simulink model "TST_Rail_SetPoint"  (R2016b)
settings: Solver=FixedStepDiscrete  StartTime=0.0  StopTime=simTime  FixedStep=sampleTime  RelTol=1e-3
values from neighbouring files (symbols this model uses):
  testCase = 1    [initTST_Rail_SetPoint_001.m]    (also in initTST_Rail_SetPoint_002.m = 2)
libraries: simulink x5, UnitTest_Lib x2
settings Model: Creator=dulinggang  LastModifiedBy=dulinggang
settings DebuggingCC: SignalRangeChecking=error

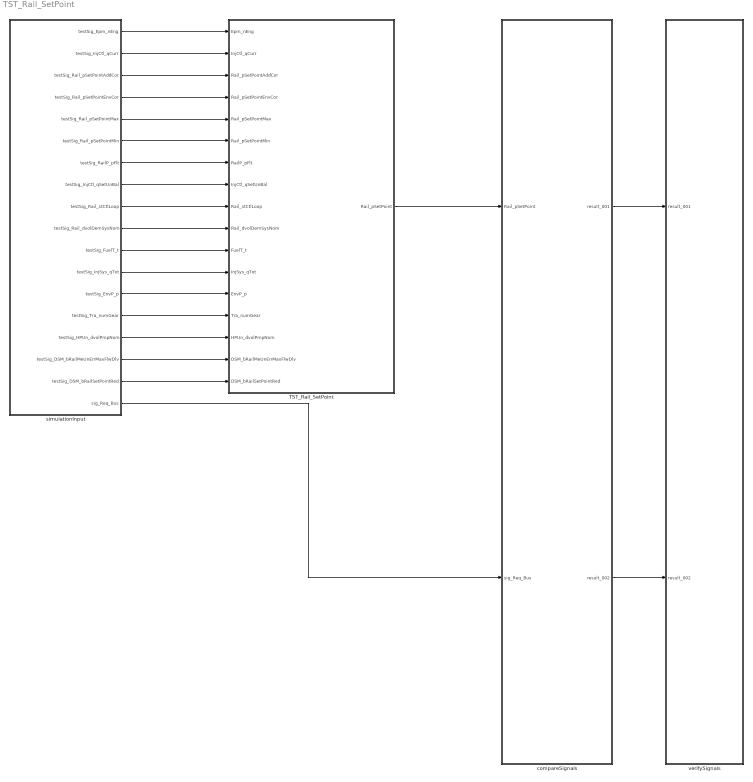
== system TST_Rail_SetPoint ==
  TST_Rail_SetPoint : Subsystem
  compareSignals : Subsystem
  simulationInput : Subsystem
  verifySignals : Subsystem
  wires:
  simulationInput/1(testSig_Epm_nEng) -> TST_Rail_SetPoint/1(Epm_nEng)
  simulationInput/2(testSig_InjCtl_qCurr) -> TST_Rail_SetPoint/2(InjCtl_qCurr)
  simulationInput/3(testSig_Rail_pSetPointAddCor) -> TST_Rail_SetPoint/3(Rail_pSetPointAddCor)
  simulationInput/4(testSig_Rail_pSetPointEnvCor) -> TST_Rail_SetPoint/4(Rail_pSetPointEnvCor)
  simulationInput/5(testSig_Rail_pSetPointMax) -> TST_Rail_SetPoint/5(Rail_pSetPointMax)
  simulationInput/6(testSig_Rail_pSetPointMin) -> TST_Rail_SetPoint/6(Rail_pSetPointMin)
  simulationInput/7(testSig_RailP_pFlt) -> TST_Rail_SetPoint/7(RailP_pFlt)
  simulationInput/8(testSig_InjCtl_qSetUnBal) -> TST_Rail_SetPoint/8(InjCtl_qSetUnBal)
  simulationInput/9(testSig_Rail_stCtlLoop) -> TST_Rail_SetPoint/9(Rail_stCtlLoop)
  simulationInput/10(testSig_Rail_dvolDemSysNom) -> TST_Rail_SetPoint/10(Rail_dvolDemSysNom)
  simulationInput/11(testSig_FuelT_t) -> TST_Rail_SetPoint/11(FuelT_t)
  simulationInput/12(testSig_InjSys_qTot) -> TST_Rail_SetPoint/12(InjSys_qTot)
  simulationInput/13(testSig_EnvP_p) -> TST_Rail_SetPoint/13(EnvP_p)
  simulationInput/14(testSig_Tra_numGear) -> TST_Rail_SetPoint/14(Tra_numGear)
  simulationInput/15(testSig_HPUn_dvolPmpNom) -> TST_Rail_SetPoint/15(HPUn_dvolPmpNom)
  simulationInput/16(testSig_DSM_bRailMeUnErrMaxFlwDlv) -> TST_Rail_SetPoint/16(DSM_bRailMeUnErrMaxFlwDlv)
  simulationInput/17(testSig_DSM_bRailSetPointRed) -> TST_Rail_SetPoint/17(DSM_bRailSetPointRed)
  TST_Rail_SetPoint/1(Rail_pSetPoint) -> compareSignals/1(Rail_pSetPoint)
  simulationInput/18(sig_Req_Bus) -> compareSignals/2(sig_Req_Bus)
  compareSignals/1(result_001) -> verifySignals/1(result_001)
  compareSignals/2(result_002) -> verifySignals/2(result_002)

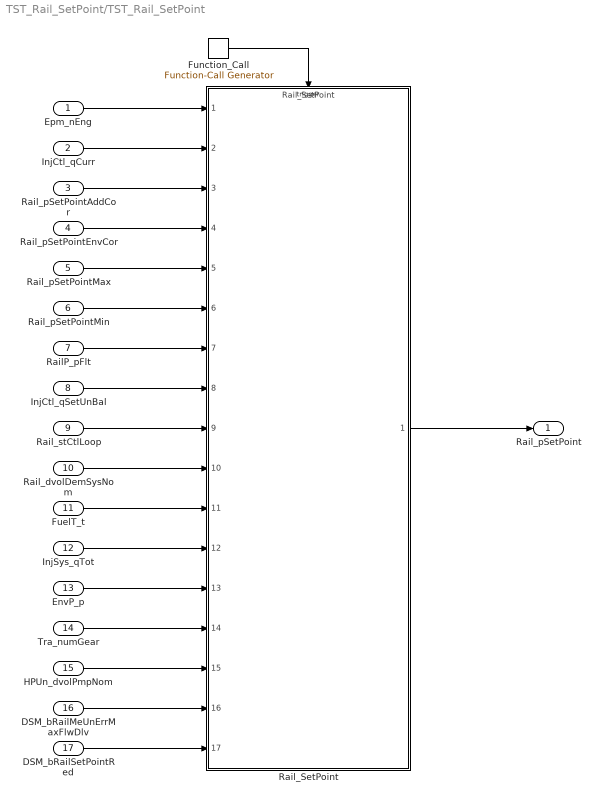
== system TST_Rail_SetPoint/TST_Rail_SetPoint ==
  Epm_nEng : Inport
  InjCtl_qCurr : Inport  Port=2
  Rail_pSetPointAddCor : Inport  Port=3
  Rail_pSetPointEnvCor : Inport  Port=4
  Rail_pSetPointMax : Inport  Port=5
  Rail_pSetPointMin : Inport  Port=6
  RailP_pFlt : Inport  Port=7
  InjCtl_qSetUnBal : Inport  Port=8
  Rail_stCtlLoop : Inport  Port=9
  Rail_dvolDemSysNom : Inport  Port=10
  FuelT_t : Inport  Port=11
  InjSys_qTot : Inport  Port=12
  EnvP_p : Inport  Port=13
  Tra_numGear : Inport  Port=14
  HPUn_dvolPmpNom : Inport  Port=15
  DSM_bRailMeUnErrMaxFlwDlv : Inport  Port=16
  DSM_bRailSetPointRed : Inport  Port=17
  Function_Call : simulink/Ports & Subsystems/Function-Call Generator  sample_time=sampleTime  numberOfIterations=1
  Rail_SetPoint : ModelReference  ModelNameDialog=Rail_SetPoint  SimulationMode=Normal  ModelReferenceVersion=1.69  TriggerPortName=function  TriggerPortTriggerType=function-call  TriggerPortStatesWhenEnabling=held
  Rail_pSetPoint : Outport
  wires:
  Function_Call/1 -> Rail_SetPoint/Trigger
  Epm_nEng/1 -> Rail_SetPoint/1
  InjCtl_qCurr/1 -> Rail_SetPoint/2
  Rail_pSetPointAddCor/1 -> Rail_SetPoint/3
  Rail_pSetPointEnvCor/1 -> Rail_SetPoint/4
  Rail_pSetPointMax/1 -> Rail_SetPoint/5
  Rail_pSetPointMin/1 -> Rail_SetPoint/6
  RailP_pFlt/1 -> Rail_SetPoint/7
  InjCtl_qSetUnBal/1 -> Rail_SetPoint/8
  Rail_stCtlLoop/1 -> Rail_SetPoint/9
  Rail_dvolDemSysNom/1 -> Rail_SetPoint/10
  FuelT_t/1 -> Rail_SetPoint/11
  InjSys_qTot/1 -> Rail_SetPoint/12
  EnvP_p/1 -> Rail_SetPoint/13
  Tra_numGear/1 -> Rail_SetPoint/14
  HPUn_dvolPmpNom/1 -> Rail_SetPoint/15
  DSM_bRailMeUnErrMaxFlwDlv/1 -> Rail_SetPoint/16
  DSM_bRailSetPointRed/1 -> Rail_SetPoint/17
  Rail_SetPoint/1 -> Rail_pSetPoint/1

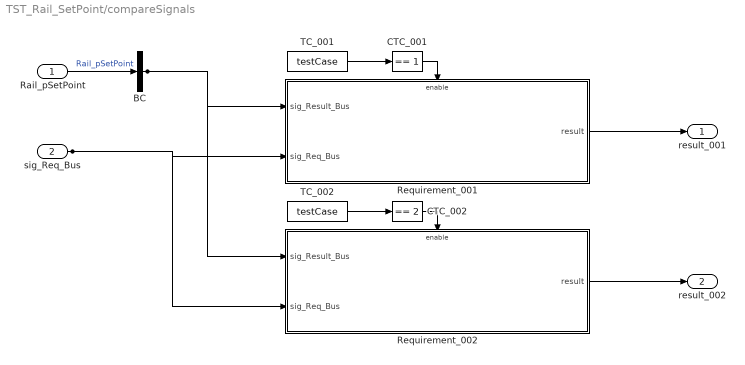
== system TST_Rail_SetPoint/compareSignals ==
  Rail_pSetPoint : Inport
  sig_Req_Bus : Inport  Port=2
  BC : BusCreator  Inputs=1
  CTC_001 : simulink/Logic and Bit Operations/Compare To Constant  relop===  const=1  OutDataTypeStr=boolean
  CTC_002 : simulink/Logic and Bit Operations/Compare To Constant  relop===  const=2  OutDataTypeStr=boolean
  Requirement_001 : Subsystem
  Requirement_002 : Subsystem
  TC_001 : Constant  Value=testCase
  TC_002 : Constant  Value=testCase
  result_001 : Outport
  result_002 : Outport  Port=2
  wires:
  Rail_pSetPoint/1 -> BC/1  "Rail_pSetPoint"
  TC_001/1 -> CTC_001/1
  CTC_001/1 -> Requirement_001/Enable
  sig_Req_Bus/1 -> Requirement_001/2(sig_Req_Bus), Requirement_002/2(sig_Req_Bus)
  BC/1 -> Requirement_001/1(sig_Result_Bus), Requirement_002/1(sig_Result_Bus)
  Requirement_001/1(result) -> result_001/1
  TC_002/1 -> CTC_002/1
  CTC_002/1 -> Requirement_002/Enable
  Requirement_002/1(result) -> result_002/1

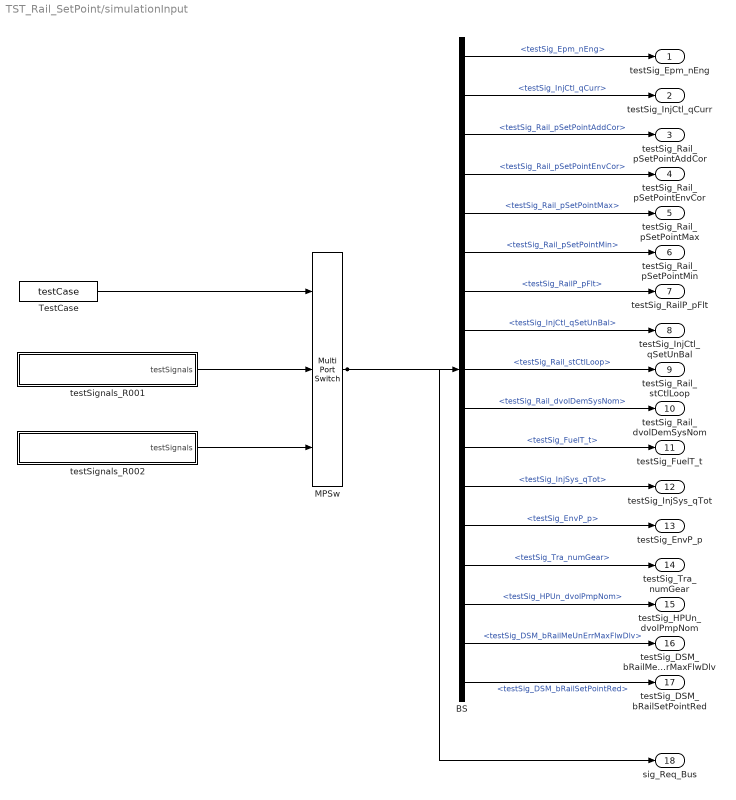
== system TST_Rail_SetPoint/simulationInput ==
  BS : BusSelector  OutputSignals=testSig_Epm_nEng,testSig_InjCtl_qCurr,testSig_Rail_pSetPointAddCor,testSig_Rail_pSetPointEnvCor,testSig_Rail_pSetPointMax,testSig_Rail_pSetPointMin,testSig_RailP_pFlt,testSig_InjCtl_qSetUnBal,testSig_Rail_stCtlLoop,testSig_Rail_dvolDemSysNom,testSig_FuelT_t,testSig_InjSys_qTot,testSig_EnvP_p,testSig_Tra_numGear,testSig_HPUn_dvolPmpNom,testSig_DSM_bRailMeUnErrMaxFlwDlv,testSig_DSM_bRailSetPointRed
  MPSw : MultiPortSwitch  Inputs=2  SaturateOnIntegerOverflow=on  InputSameDT=on
  TestCase : Constant  Value=testCase
  testSignals_R001 : Subsystem
  testSignals_R002 : Subsystem
  testSig_Epm_nEng : Outport
  testSig_InjCtl_qCurr : Outport  Port=2
  testSig_Rail_pSetPointAddCor : Outport  Port=3
  testSig_Rail_pSetPointEnvCor : Outport  Port=4
  testSig_Rail_pSetPointMax : Outport  Port=5
  testSig_Rail_pSetPointMin : Outport  Port=6
  testSig_RailP_pFlt : Outport  Port=7
  testSig_InjCtl_qSetUnBal : Outport  Port=8
  testSig_Rail_stCtlLoop : Outport  Port=9
  testSig_Rail_dvolDemSysNom : Outport  Port=10
  testSig_FuelT_t : Outport  Port=11
  testSig_InjSys_qTot : Outport  Port=12
  testSig_EnvP_p : Outport  Port=13
  testSig_Tra_numGear : Outport  Port=14
  testSig_HPUn_dvolPmpNom : Outport  Port=15
  testSig_DSM_bRailMeUnErrMaxFlwDlv : Outport  Port=16
  testSig_DSM_bRailSetPointRed : Outport  Port=17
  sig_Req_Bus : Outport  Port=18
  wires:
  BS/1 -> testSig_Epm_nEng/1  "<testSig_Epm_nEng>"
  BS/2 -> testSig_InjCtl_qCurr/1  "<testSig_InjCtl_qCurr>"
  BS/3 -> testSig_Rail_pSetPointAddCor/1  "<testSig_Rail_pSetPointAddCor>"
  BS/4 -> testSig_Rail_pSetPointEnvCor/1  "<testSig_Rail_pSetPointEnvCor>"
  BS/5 -> testSig_Rail_pSetPointMax/1  "<testSig_Rail_pSetPointMax>"
  BS/6 -> testSig_Rail_pSetPointMin/1  "<testSig_Rail_pSetPointMin>"
  BS/7 -> testSig_RailP_pFlt/1  "<testSig_RailP_pFlt>"
  BS/8 -> testSig_InjCtl_qSetUnBal/1  "<testSig_InjCtl_qSetUnBal>"
  BS/9 -> testSig_Rail_stCtlLoop/1  "<testSig_Rail_stCtlLoop>"
  BS/10 -> testSig_Rail_dvolDemSysNom/1  "<testSig_Rail_dvolDemSysNom>"
  BS/11 -> testSig_FuelT_t/1  "<testSig_FuelT_t>"
  BS/12 -> testSig_InjSys_qTot/1  "<testSig_InjSys_qTot>"
  BS/13 -> testSig_EnvP_p/1  "<testSig_EnvP_p>"
  BS/14 -> testSig_Tra_numGear/1  "<testSig_Tra_numGear>"
  BS/15 -> testSig_HPUn_dvolPmpNom/1  "<testSig_HPUn_dvolPmpNom>"
  BS/16 -> testSig_DSM_bRailMeUnErrMaxFlwDlv/1  "<testSig_DSM_bRailMeUnErrMaxFlwDlv>"
  BS/17 -> testSig_DSM_bRailSetPointRed/1  "<testSig_DSM_bRailSetPointRed>"
  MPSw/1 -> BS/1, sig_Req_Bus/1
  TestCase/1 -> MPSw/1
  testSignals_R001/1(testSignals) -> MPSw/2
  testSignals_R002/1(testSignals) -> MPSw/3

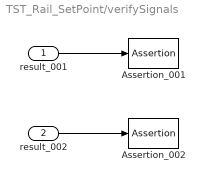
== system TST_Rail_SetPoint/verifySignals ==
  result_001 : Inport
  result_002 : Inport  Port=2
  Assertion_001 : Assertion  Enabled=off
  Assertion_002 : Assertion  Enabled=off
  wires:
  result_001/1 -> Assertion_001/1
  result_002/1 -> Assertion_002/1

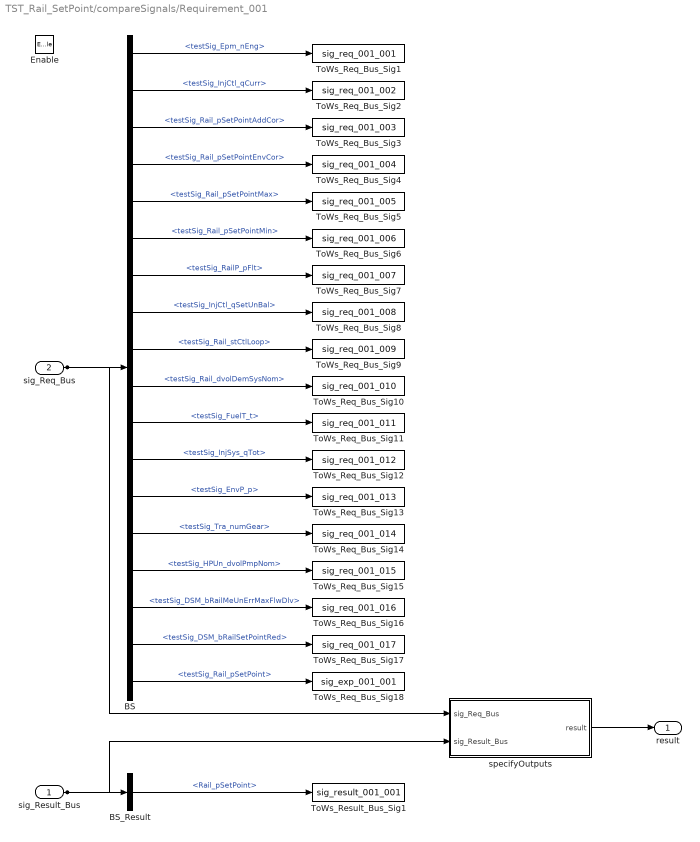
== system TST_Rail_SetPoint/compareSignals/Requirement_001 ==
  sig_Result_Bus : Inport
  sig_Req_Bus : Inport  Port=2
  Enable : EnablePort
  BS : BusSelector  OutputSignals=testSig_Epm_nEng,testSig_InjCtl_qCurr,testSig_Rail_pSetPointAddCor,testSig_Rail_pSetPointEnvCor,testSig_Rail_pSetPointMax,testSig_Rail_pSetPointMin,testSig_RailP_pFlt,testSig_InjCtl_qSetUnBal,testSig_Rail_stCtlLoop,testSig_Rail_dvolDemSysNom,testSig_FuelT_t,testSig_InjSys_qTot,testSig_EnvP_p,testSig_Tra_numGear,testSig_HPUn_dvolPmpNom,testSig_DSM_bRailMeUnErrMaxFlwDlv,testSig_DSM_bRailSetPointRed,testSig_Rail_pSetPoint
  BS_Result : BusSelector  OutputSignals=Rail_pSetPoint
  ToWs_Req_Bus_Sig1 : ToWorkspace  VariableName=sig_req_001_001  SaveFormat=Structure With Time
  ToWs_Req_Bus_Sig10 : ToWorkspace  VariableName=sig_req_001_010  SaveFormat=Structure With Time
  ToWs_Req_Bus_Sig11 : ToWorkspace  VariableName=sig_req_001_011  SaveFormat=Structure With Time
  ToWs_Req_Bus_Sig12 : ToWorkspace  VariableName=sig_req_001_012  SaveFormat=Structure With Time
  ToWs_Req_Bus_Sig13 : ToWorkspace  VariableName=sig_req_001_013  SaveFormat=Structure With Time
  ToWs_Req_Bus_Sig14 : ToWorkspace  VariableName=sig_req_001_014  SaveFormat=Structure With Time
  ToWs_Req_Bus_Sig15 : ToWorkspace  VariableName=sig_req_001_015  SaveFormat=Structure With Time
  ToWs_Req_Bus_Sig16 : ToWorkspace  VariableName=sig_req_001_016  SaveFormat=Structure With Time
  ToWs_Req_Bus_Sig17 : ToWorkspace  VariableName=sig_req_001_017  SaveFormat=Structure With Time
  ToWs_Req_Bus_Sig18 : ToWorkspace  VariableName=sig_exp_001_001  SaveFormat=Structure With Time
  ToWs_Req_Bus_Sig2 : ToWorkspace  VariableName=sig_req_001_002  SaveFormat=Structure With Time
  ToWs_Req_Bus_Sig3 : ToWorkspace  VariableName=sig_req_001_003  SaveFormat=Structure With Time
  ToWs_Req_Bus_Sig4 : ToWorkspace  VariableName=sig_req_001_004  SaveFormat=Structure With Time
  ToWs_Req_Bus_Sig5 : ToWorkspace  VariableName=sig_req_001_005  SaveFormat=Structure With Time
  ToWs_Req_Bus_Sig6 : ToWorkspace  VariableName=sig_req_001_006  SaveFormat=Structure With Time
  ToWs_Req_Bus_Sig7 : ToWorkspace  VariableName=sig_req_001_007  SaveFormat=Structure With Time
  ToWs_Req_Bus_Sig8 : ToWorkspace  VariableName=sig_req_001_008  SaveFormat=Structure With Time
  ToWs_Req_Bus_Sig9 : ToWorkspace  VariableName=sig_req_001_009  SaveFormat=Structure With Time
  ToWs_Result_Bus_Sig1 : ToWorkspace  VariableName=sig_result_001_001  SaveFormat=Structure With Time
  specifyOutputs : Subsystem
  result : Outport
  wires:
  sig_Req_Bus/1 -> BS/1, specifyOutputs/1(sig_Req_Bus)
  BS/1 -> ToWs_Req_Bus_Sig1/1  "<testSig_Epm_nEng>"
  BS/2 -> ToWs_Req_Bus_Sig2/1  "<testSig_InjCtl_qCurr>"
  BS/3 -> ToWs_Req_Bus_Sig3/1  "<testSig_Rail_pSetPointAddCor>"
  BS/4 -> ToWs_Req_Bus_Sig4/1  "<testSig_Rail_pSetPointEnvCor>"
  BS/5 -> ToWs_Req_Bus_Sig5/1  "<testSig_Rail_pSetPointMax>"
  BS/6 -> ToWs_Req_Bus_Sig6/1  "<testSig_Rail_pSetPointMin>"
  BS/7 -> ToWs_Req_Bus_Sig7/1  "<testSig_RailP_pFlt>"
  BS/8 -> ToWs_Req_Bus_Sig8/1  "<testSig_InjCtl_qSetUnBal>"
  BS/9 -> ToWs_Req_Bus_Sig9/1  "<testSig_Rail_stCtlLoop>"
  BS/10 -> ToWs_Req_Bus_Sig10/1  "<testSig_Rail_dvolDemSysNom>"
  BS/11 -> ToWs_Req_Bus_Sig11/1  "<testSig_FuelT_t>"
  BS/12 -> ToWs_Req_Bus_Sig12/1  "<testSig_InjSys_qTot>"
  BS/13 -> ToWs_Req_Bus_Sig13/1  "<testSig_EnvP_p>"
  BS/14 -> ToWs_Req_Bus_Sig14/1  "<testSig_Tra_numGear>"
  BS/15 -> ToWs_Req_Bus_Sig15/1  "<testSig_HPUn_dvolPmpNom>"
  BS/16 -> ToWs_Req_Bus_Sig16/1  "<testSig_DSM_bRailMeUnErrMaxFlwDlv>"
  BS/17 -> ToWs_Req_Bus_Sig17/1  "<testSig_DSM_bRailSetPointRed>"
  BS/18 -> ToWs_Req_Bus_Sig18/1  "<testSig_Rail_pSetPoint>"
  sig_Result_Bus/1 -> BS_Result/1, specifyOutputs/2(sig_Result_Bus)
  BS_Result/1 -> ToWs_Result_Bus_Sig1/1  "<Rail_pSetPoint>"
  specifyOutputs/1(result) -> result/1

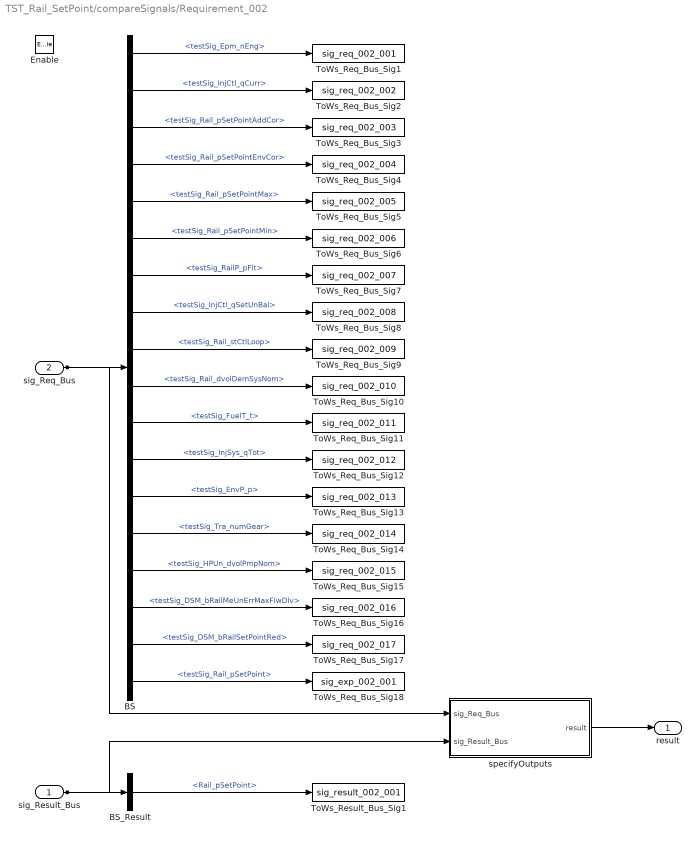
== system TST_Rail_SetPoint/compareSignals/Requirement_002 ==
  sig_Result_Bus : Inport
  sig_Req_Bus : Inport  Port=2
  Enable : EnablePort
  BS : BusSelector  OutputSignals=testSig_Epm_nEng,testSig_InjCtl_qCurr,testSig_Rail_pSetPointAddCor,testSig_Rail_pSetPointEnvCor,testSig_Rail_pSetPointMax,testSig_Rail_pSetPointMin,testSig_RailP_pFlt,testSig_InjCtl_qSetUnBal,testSig_Rail_stCtlLoop,testSig_Rail_dvolDemSysNom,testSig_FuelT_t,testSig_InjSys_qTot,testSig_EnvP_p,testSig_Tra_numGear,testSig_HPUn_dvolPmpNom,testSig_DSM_bRailMeUnErrMaxFlwDlv,testSig_DSM_bRailSetPointRed,testSig_Rail_pSetPoint
  BS_Result : BusSelector  OutputSignals=Rail_pSetPoint
  ToWs_Req_Bus_Sig1 : ToWorkspace  VariableName=sig_req_002_001  SaveFormat=Structure With Time
  ToWs_Req_Bus_Sig10 : ToWorkspace  VariableName=sig_req_002_010  SaveFormat=Structure With Time
  ToWs_Req_Bus_Sig11 : ToWorkspace  VariableName=sig_req_002_011  SaveFormat=Structure With Time
  ToWs_Req_Bus_Sig12 : ToWorkspace  VariableName=sig_req_002_012  SaveFormat=Structure With Time
  ToWs_Req_Bus_Sig13 : ToWorkspace  VariableName=sig_req_002_013  SaveFormat=Structure With Time
  ToWs_Req_Bus_Sig14 : ToWorkspace  VariableName=sig_req_002_014  SaveFormat=Structure With Time
  ToWs_Req_Bus_Sig15 : ToWorkspace  VariableName=sig_req_002_015  SaveFormat=Structure With Time
  ToWs_Req_Bus_Sig16 : ToWorkspace  VariableName=sig_req_002_016  SaveFormat=Structure With Time
  ToWs_Req_Bus_Sig17 : ToWorkspace  VariableName=sig_req_002_017  SaveFormat=Structure With Time
  ToWs_Req_Bus_Sig18 : ToWorkspace  VariableName=sig_exp_002_001  SaveFormat=Structure With Time
  ToWs_Req_Bus_Sig2 : ToWorkspace  VariableName=sig_req_002_002  SaveFormat=Structure With Time
  ToWs_Req_Bus_Sig3 : ToWorkspace  VariableName=sig_req_002_003  SaveFormat=Structure With Time
  ToWs_Req_Bus_Sig4 : ToWorkspace  VariableName=sig_req_002_004  SaveFormat=Structure With Time
  ToWs_Req_Bus_Sig5 : ToWorkspace  VariableName=sig_req_002_005  SaveFormat=Structure With Time
  ToWs_Req_Bus_Sig6 : ToWorkspace  VariableName=sig_req_002_006  SaveFormat=Structure With Time
  ToWs_Req_Bus_Sig7 : ToWorkspace  VariableName=sig_req_002_007  SaveFormat=Structure With Time
  ToWs_Req_Bus_Sig8 : ToWorkspace  VariableName=sig_req_002_008  SaveFormat=Structure With Time
  ToWs_Req_Bus_Sig9 : ToWorkspace  VariableName=sig_req_002_009  SaveFormat=Structure With Time
  ToWs_Result_Bus_Sig1 : ToWorkspace  VariableName=sig_result_002_001  SaveFormat=Structure With Time
  specifyOutputs : Subsystem
  result : Outport
  wires:
  sig_Req_Bus/1 -> BS/1, specifyOutputs/1(sig_Req_Bus)
  BS/1 -> ToWs_Req_Bus_Sig1/1  "<testSig_Epm_nEng>"
  BS/2 -> ToWs_Req_Bus_Sig2/1  "<testSig_InjCtl_qCurr>"
  BS/3 -> ToWs_Req_Bus_Sig3/1  "<testSig_Rail_pSetPointAddCor>"
  BS/4 -> ToWs_Req_Bus_Sig4/1  "<testSig_Rail_pSetPointEnvCor>"
  BS/5 -> ToWs_Req_Bus_Sig5/1  "<testSig_Rail_pSetPointMax>"
  BS/6 -> ToWs_Req_Bus_Sig6/1  "<testSig_Rail_pSetPointMin>"
  BS/7 -> ToWs_Req_Bus_Sig7/1  "<testSig_RailP_pFlt>"
  BS/8 -> ToWs_Req_Bus_Sig8/1  "<testSig_InjCtl_qSetUnBal>"
  BS/9 -> ToWs_Req_Bus_Sig9/1  "<testSig_Rail_stCtlLoop>"
  BS/10 -> ToWs_Req_Bus_Sig10/1  "<testSig_Rail_dvolDemSysNom>"
  BS/11 -> ToWs_Req_Bus_Sig11/1  "<testSig_FuelT_t>"
  BS/12 -> ToWs_Req_Bus_Sig12/1  "<testSig_InjSys_qTot>"
  BS/13 -> ToWs_Req_Bus_Sig13/1  "<testSig_EnvP_p>"
  BS/14 -> ToWs_Req_Bus_Sig14/1  "<testSig_Tra_numGear>"
  BS/15 -> ToWs_Req_Bus_Sig15/1  "<testSig_HPUn_dvolPmpNom>"
  BS/16 -> ToWs_Req_Bus_Sig16/1  "<testSig_DSM_bRailMeUnErrMaxFlwDlv>"
  BS/17 -> ToWs_Req_Bus_Sig17/1  "<testSig_DSM_bRailSetPointRed>"
  BS/18 -> ToWs_Req_Bus_Sig18/1  "<testSig_Rail_pSetPoint>"
  sig_Result_Bus/1 -> BS_Result/1, specifyOutputs/2(sig_Result_Bus)
  BS_Result/1 -> ToWs_Result_Bus_Sig1/1  "<Rail_pSetPoint>"
  specifyOutputs/1(result) -> result/1

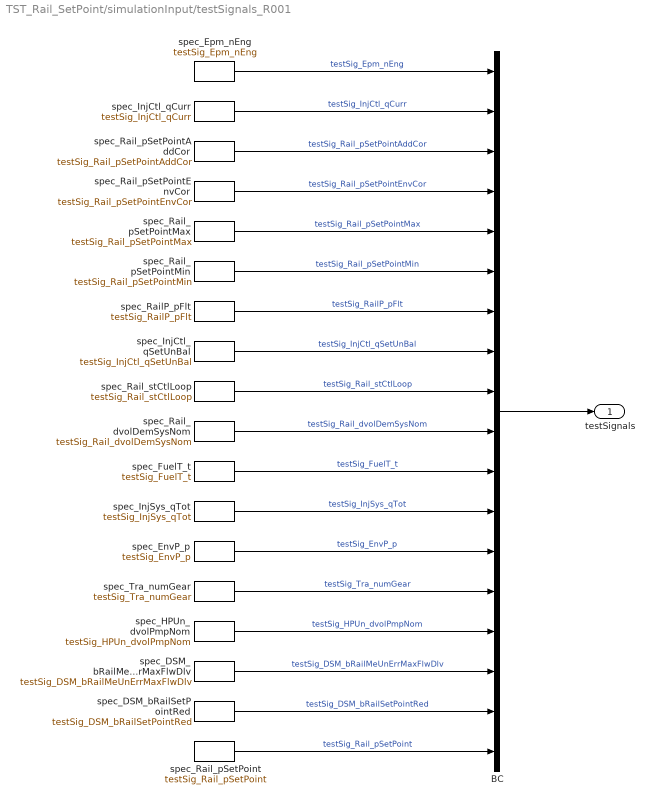
== system TST_Rail_SetPoint/simulationInput/testSignals_R001 ==
  BC : BusCreator  Inputs=18
  spec_DSM_bRailMeUnErrMaxFlwDlv : FromWorkspace  VariableName=testSig_DSM_bRailMeUnErrMaxFlwDlv  Interpolate=off  OutputAfterFinalValue=Holding final value
  spec_DSM_bRailSetPointRed : FromWorkspace  VariableName=testSig_DSM_bRailSetPointRed  Interpolate=off  OutputAfterFinalValue=Holding final value
  spec_EnvP_p : FromWorkspace  VariableName=testSig_EnvP_p  Interpolate=off  OutputAfterFinalValue=Holding final value
  spec_Epm_nEng : FromWorkspace  VariableName=testSig_Epm_nEng  Interpolate=off  OutputAfterFinalValue=Holding final value
  spec_FuelT_t : FromWorkspace  VariableName=testSig_FuelT_t  Interpolate=off  OutputAfterFinalValue=Holding final value
  spec_HPUn_dvolPmpNom : FromWorkspace  VariableName=testSig_HPUn_dvolPmpNom  Interpolate=off  OutputAfterFinalValue=Holding final value
  spec_InjCtl_qCurr : FromWorkspace  VariableName=testSig_InjCtl_qCurr  Interpolate=off  OutputAfterFinalValue=Holding final value
  spec_InjCtl_qSetUnBal : FromWorkspace  VariableName=testSig_InjCtl_qSetUnBal  Interpolate=off  OutputAfterFinalValue=Holding final value
  spec_InjSys_qTot : FromWorkspace  VariableName=testSig_InjSys_qTot  Interpolate=off  OutputAfterFinalValue=Holding final value
  spec_RailP_pFlt : FromWorkspace  VariableName=testSig_RailP_pFlt  Interpolate=off  OutputAfterFinalValue=Holding final value
  spec_Rail_dvolDemSysNom : FromWorkspace  VariableName=testSig_Rail_dvolDemSysNom  Interpolate=off  OutputAfterFinalValue=Holding final value
  spec_Rail_pSetPoint : FromWorkspace  VariableName=testSig_Rail_pSetPoint  Interpolate=off  OutputAfterFinalValue=Holding final value
  spec_Rail_pSetPointAddCor : FromWorkspace  VariableName=testSig_Rail_pSetPointAddCor  Interpolate=off  OutputAfterFinalValue=Holding final value
  spec_Rail_pSetPointEnvCor : FromWorkspace  VariableName=testSig_Rail_pSetPointEnvCor  Interpolate=off  OutputAfterFinalValue=Holding final value
  spec_Rail_pSetPointMax : FromWorkspace  VariableName=testSig_Rail_pSetPointMax  Interpolate=off  OutputAfterFinalValue=Holding final value
  spec_Rail_pSetPointMin : FromWorkspace  VariableName=testSig_Rail_pSetPointMin  Interpolate=off  OutputAfterFinalValue=Holding final value
  spec_Rail_stCtlLoop : FromWorkspace  VariableName=testSig_Rail_stCtlLoop  Interpolate=off  OutputAfterFinalValue=Holding final value
  spec_Tra_numGear : FromWorkspace  VariableName=testSig_Tra_numGear  Interpolate=off  OutputAfterFinalValue=Holding final value
  testSignals : Outport
  wires:
  BC/1 -> testSignals/1
  spec_Epm_nEng/1 -> BC/1  "testSig_Epm_nEng"
  spec_InjCtl_qCurr/1 -> BC/2  "testSig_InjCtl_qCurr"
  spec_Rail_pSetPointAddCor/1 -> BC/3  "testSig_Rail_pSetPointAddCor"
  spec_Rail_pSetPointEnvCor/1 -> BC/4  "testSig_Rail_pSetPointEnvCor"
  spec_Rail_pSetPointMax/1 -> BC/5  "testSig_Rail_pSetPointMax"
  spec_Rail_pSetPointMin/1 -> BC/6  "testSig_Rail_pSetPointMin"
  spec_RailP_pFlt/1 -> BC/7  "testSig_RailP_pFlt"
  spec_InjCtl_qSetUnBal/1 -> BC/8  "testSig_InjCtl_qSetUnBal"
  spec_Rail_stCtlLoop/1 -> BC/9  "testSig_Rail_stCtlLoop"
  spec_Rail_dvolDemSysNom/1 -> BC/10  "testSig_Rail_dvolDemSysNom"
  spec_FuelT_t/1 -> BC/11  "testSig_FuelT_t"
  spec_InjSys_qTot/1 -> BC/12  "testSig_InjSys_qTot"
  spec_EnvP_p/1 -> BC/13  "testSig_EnvP_p"
  spec_Tra_numGear/1 -> BC/14  "testSig_Tra_numGear"
  spec_HPUn_dvolPmpNom/1 -> BC/15  "testSig_HPUn_dvolPmpNom"
  spec_DSM_bRailMeUnErrMaxFlwDlv/1 -> BC/16  "testSig_DSM_bRailMeUnErrMaxFlwDlv"
  spec_DSM_bRailSetPointRed/1 -> BC/17  "testSig_DSM_bRailSetPointRed"
  spec_Rail_pSetPoint/1 -> BC/18  "testSig_Rail_pSetPoint"

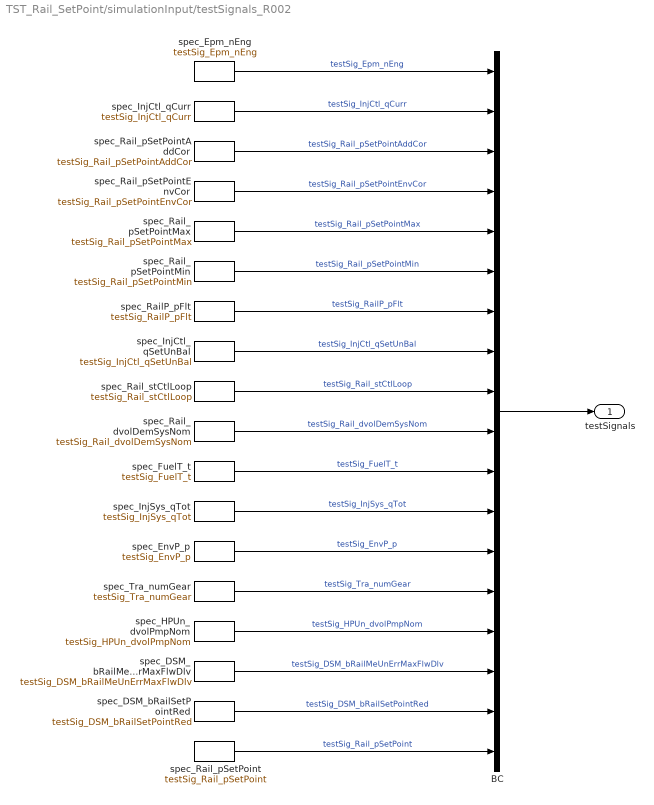
== system TST_Rail_SetPoint/simulationInput/testSignals_R002 ==
  BC : BusCreator  Inputs=18
  spec_DSM_bRailMeUnErrMaxFlwDlv : FromWorkspace  VariableName=testSig_DSM_bRailMeUnErrMaxFlwDlv  Interpolate=off  OutputAfterFinalValue=Holding final value
  spec_DSM_bRailSetPointRed : FromWorkspace  VariableName=testSig_DSM_bRailSetPointRed  Interpolate=off  OutputAfterFinalValue=Holding final value
  spec_EnvP_p : FromWorkspace  VariableName=testSig_EnvP_p  Interpolate=off  OutputAfterFinalValue=Holding final value
  spec_Epm_nEng : FromWorkspace  VariableName=testSig_Epm_nEng  Interpolate=off  OutputAfterFinalValue=Holding final value
  spec_FuelT_t : FromWorkspace  VariableName=testSig_FuelT_t  Interpolate=off  OutputAfterFinalValue=Holding final value
  spec_HPUn_dvolPmpNom : FromWorkspace  VariableName=testSig_HPUn_dvolPmpNom  Interpolate=off  OutputAfterFinalValue=Holding final value
  spec_InjCtl_qCurr : FromWorkspace  VariableName=testSig_InjCtl_qCurr  Interpolate=off  OutputAfterFinalValue=Holding final value
  spec_InjCtl_qSetUnBal : FromWorkspace  VariableName=testSig_InjCtl_qSetUnBal  Interpolate=off  OutputAfterFinalValue=Holding final value
  spec_InjSys_qTot : FromWorkspace  VariableName=testSig_InjSys_qTot  Interpolate=off  OutputAfterFinalValue=Holding final value
  spec_RailP_pFlt : FromWorkspace  VariableName=testSig_RailP_pFlt  Interpolate=off  OutputAfterFinalValue=Holding final value
  spec_Rail_dvolDemSysNom : FromWorkspace  VariableName=testSig_Rail_dvolDemSysNom  Interpolate=off  OutputAfterFinalValue=Holding final value
  spec_Rail_pSetPoint : FromWorkspace  VariableName=testSig_Rail_pSetPoint  Interpolate=off  OutputAfterFinalValue=Holding final value
  spec_Rail_pSetPointAddCor : FromWorkspace  VariableName=testSig_Rail_pSetPointAddCor  Interpolate=off  OutputAfterFinalValue=Holding final value
  spec_Rail_pSetPointEnvCor : FromWorkspace  VariableName=testSig_Rail_pSetPointEnvCor  Interpolate=off  OutputAfterFinalValue=Holding final value
  spec_Rail_pSetPointMax : FromWorkspace  VariableName=testSig_Rail_pSetPointMax  Interpolate=off  OutputAfterFinalValue=Holding final value
  spec_Rail_pSetPointMin : FromWorkspace  VariableName=testSig_Rail_pSetPointMin  Interpolate=off  OutputAfterFinalValue=Holding final value
  spec_Rail_stCtlLoop : FromWorkspace  VariableName=testSig_Rail_stCtlLoop  Interpolate=off  OutputAfterFinalValue=Holding final value
  spec_Tra_numGear : FromWorkspace  VariableName=testSig_Tra_numGear  Interpolate=off  OutputAfterFinalValue=Holding final value
  testSignals : Outport
  wires:
  BC/1 -> testSignals/1
  spec_Epm_nEng/1 -> BC/1  "testSig_Epm_nEng"
  spec_InjCtl_qCurr/1 -> BC/2  "testSig_InjCtl_qCurr"
  spec_Rail_pSetPointAddCor/1 -> BC/3  "testSig_Rail_pSetPointAddCor"
  spec_Rail_pSetPointEnvCor/1 -> BC/4  "testSig_Rail_pSetPointEnvCor"
  spec_Rail_pSetPointMax/1 -> BC/5  "testSig_Rail_pSetPointMax"
  spec_Rail_pSetPointMin/1 -> BC/6  "testSig_Rail_pSetPointMin"
  spec_RailP_pFlt/1 -> BC/7  "testSig_RailP_pFlt"
  spec_InjCtl_qSetUnBal/1 -> BC/8  "testSig_InjCtl_qSetUnBal"
  spec_Rail_stCtlLoop/1 -> BC/9  "testSig_Rail_stCtlLoop"
  spec_Rail_dvolDemSysNom/1 -> BC/10  "testSig_Rail_dvolDemSysNom"
  spec_FuelT_t/1 -> BC/11  "testSig_FuelT_t"
  spec_InjSys_qTot/1 -> BC/12  "testSig_InjSys_qTot"
  spec_EnvP_p/1 -> BC/13  "testSig_EnvP_p"
  spec_Tra_numGear/1 -> BC/14  "testSig_Tra_numGear"
  spec_HPUn_dvolPmpNom/1 -> BC/15  "testSig_HPUn_dvolPmpNom"
  spec_DSM_bRailMeUnErrMaxFlwDlv/1 -> BC/16  "testSig_DSM_bRailMeUnErrMaxFlwDlv"
  spec_DSM_bRailSetPointRed/1 -> BC/17  "testSig_DSM_bRailSetPointRed"
  spec_Rail_pSetPoint/1 -> BC/18  "testSig_Rail_pSetPoint"

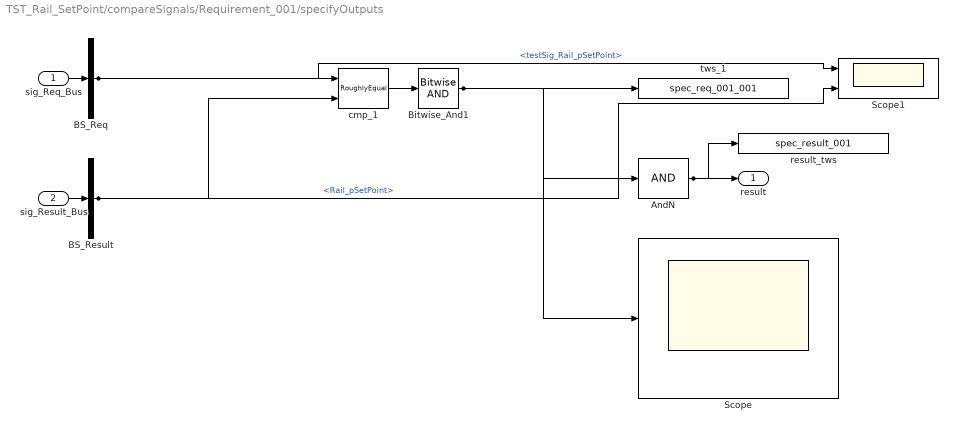
== system TST_Rail_SetPoint/compareSignals/Requirement_001/specifyOutputs ==
  sig_Req_Bus : Inport
  sig_Result_Bus : Inport  Port=2
  AndN : Logic  Inputs=1
  BS_Req : BusSelector  OutputSignals=testSig_Rail_pSetPoint
  BS_Result : BusSelector  OutputSignals=Rail_pSetPoint
  Bitwise_And1 : simulink/Logic and Bit Operations/Bitwise Operator  logicop=AND  UseBitMask=off  BitMask=bin2dec('11011001')  BitMaskRealWorld=Stored Integer
  Scope : Scope
  Scope1 : Scope  NumInputPorts=2
  cmp_1 : UnitTest_Lib/RoughlyEqual  slope=0.1
  result_tws : ToWorkspace  VariableName=spec_result_001
  tws_1 : ToWorkspace  VariableName=spec_req_001_001
  result : Outport
  wires:
  sig_Req_Bus/1 -> BS_Req/1
  sig_Result_Bus/1 -> BS_Result/1
  AndN/1 -> result/1, result_tws/1
  BS_Req/1 -> cmp_1/1, Scope1/1  "<testSig_Rail_pSetPoint>"
  BS_Result/1 -> cmp_1/2, Scope1/2  "<Rail_pSetPoint>"
  cmp_1/1 -> Bitwise_And1/1
  Bitwise_And1/1 -> tws_1/1, AndN/1, Scope/1

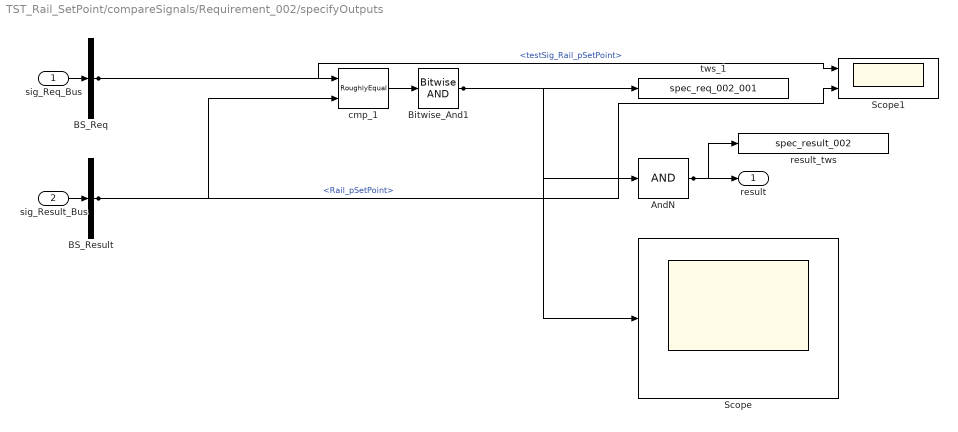
== system TST_Rail_SetPoint/compareSignals/Requirement_002/specifyOutputs ==
  sig_Req_Bus : Inport
  sig_Result_Bus : Inport  Port=2
  AndN : Logic  Inputs=1
  BS_Req : BusSelector  OutputSignals=testSig_Rail_pSetPoint
  BS_Result : BusSelector  OutputSignals=Rail_pSetPoint
  Bitwise_And1 : simulink/Logic and Bit Operations/Bitwise Operator  logicop=AND  UseBitMask=off  BitMask=bin2dec('11011001')  BitMaskRealWorld=Stored Integer
  Scope : Scope
  Scope1 : Scope  NumInputPorts=2
  cmp_1 : UnitTest_Lib/RoughlyEqual  slope=0.1
  result_tws : ToWorkspace  VariableName=spec_result_002
  tws_1 : ToWorkspace  VariableName=spec_req_002_001
  result : Outport
  wires:
  sig_Req_Bus/1 -> BS_Req/1
  sig_Result_Bus/1 -> BS_Result/1
  AndN/1 -> result/1, result_tws/1
  BS_Req/1 -> cmp_1/1, Scope1/1  "<testSig_Rail_pSetPoint>"
  BS_Result/1 -> cmp_1/2, Scope1/2  "<Rail_pSetPoint>"
  cmp_1/1 -> Bitwise_And1/1
  Bitwise_And1/1 -> tws_1/1, AndN/1, Scope/1
